simulink model "invpend_NL_PID"  (R2023b)
settings: Solver=VariableStepAuto  StartTime=0.0  StopTime=10.0  MaxStep=0.01  RelTol=1e-3
libraries: slpidlib x1
settings Model: Creator=bwang-ccny  LastModifiedBy=bwang-ccny

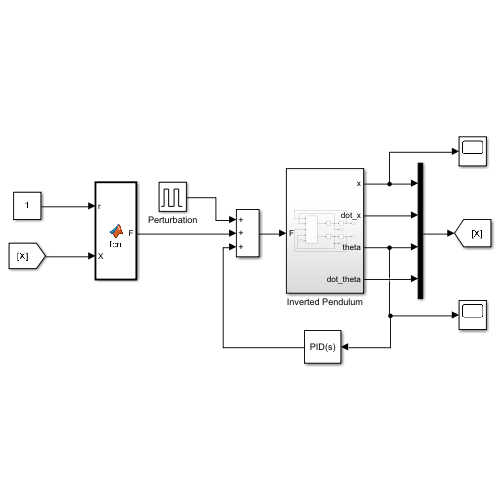
[thumbnail: Simulink's stored preview of the top-level diagram]
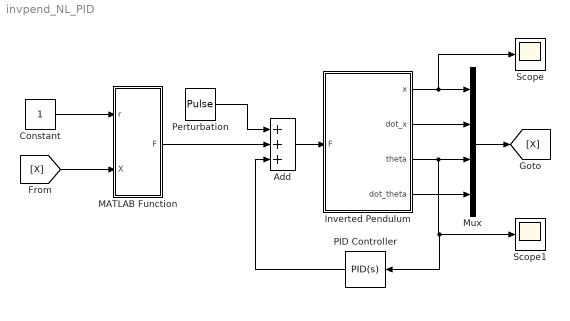
== system invpend_NL_PID ==
  Add : Sum  Inputs=+++
  Constant : Constant
  Inverted Pendulum : Subsystem
  MATLAB Function : MATLAB Function  TreatAsAtomicUnit=on
  Mux : Mux
  PID Controller : slpidlib/PID Controller  Controller=PID  Form=Parallel  TimeDomain=Continuous-time  UseExternalTs=off  SampleTime=-1  IntegratorMethod=Forward Euler  FilterMethod=Forward Euler  ControllerParametersSource=internal  P=20  I=0  UseKiTs=off  D=2  N=100  UseFilter=on  TunerSelectOption=Transfer Function Based (PID Tuner App)  InitialConditionSource=internal  InitialConditionForIntegrator=0  InitialConditionForFilter=0  DifferentiatorICPrevScaledInput=0  ExternalReset=none  TrackingMode=off  Kt=1  LimitOutput=off  SatLimitsSource=internal  UpperSaturationLimit=inf  LowerSaturationLimit=-inf  LinearizeAsGain=on  AntiWindupMode=none  Kb=1  LimitIntegrator=off  UpperIntegratorSaturationLimit=inf  LowerIntegratorSaturationLimit=-inf  POutMin=[]  POutMax=[]  IOutMin=[]  IOutMax=[]  DOutMin=[]  DOutMax=[]  NOutMin=[]  NOutMax=[]  SumOutMin=[]  SumOutMax=[]  SaturationOutMin=[]  SaturationOutMax=[]  PParamMin=[]  PParamMax=[]  IParamMin=[]  IParamMax=[]  DParamMin=[]  DParamMax=[]  NParamMin=[]  NParamMax=[]  KbParamMin=[]  KbParamMax=[]  KtParamMin=[]  KtParamMax=[]  KbOutMin=[]  KbOutMax=[]  KtOutMin=[]  KtOutMax=[]  IntegratorOutMin=[]  IntegratorOutMax=[]  FilterOutMin=[]  FilterOutMax=[]  SumI1OutMin=[]  SumI1OutMax=[]  SumI2OutMin=[]  SumI2OutMax=[]  SumI3OutMin=[]  SumI3OutMax=[]  SumI4OutMin=[]  SumI4OutMax=[]  SumDOutMin=[]  SumDOutMax=[]  DifferentiatorOutMin=[]  DifferentiatorOutMax=[]  FilterDiffOutCoefMin=[]  FilterDiffOutCoefMax=[]  ReciprocalOutMin=[]  ReciprocalOutMax=[]  SumDenOutMin=[]  SumDenOutMax=[]  SumNumOutMin=[]  SumNumOutMax=[]  DivideOutMin=[]  DivideOutMax=[]  UdiffTsProdOutMin=[]  UdiffTsProdOutMax=[]  NTsProdOutMin=[]  NTsProdOutMax=[]  UintegralTsProdOutMin=[]  UintegralTsProdOutMax=[]  UngainTsProdOutMin=[]  UngainTsProdOutMax=[]  ClampingZeroOutDataTypeStr=Inherit: Inherit via back propagation  ClampingZeroOutMin=[]  ClampingZeroOutMax=[]  FilterDenConstantOutDataTypeStr=Inherit: Inherit via back propagation  FilterDenConstantOutMin=[]  FilterDenConstantOutMax=[]  PCopyOutDataTypeStr=Inherit: Inherit via back propagation  PCopyOutMin=[]  PCopyOutMax=[]  NCopyOutDataTypeStr=Inherit: Inherit via back propagation  NCopyOutMin=[]  NCopyOutMax=[]  IntegratorContinuousStateAttributes=''  IntegratorStateMustResolveToSignalObject=off  IntegratorRTWStateStorageClass=Auto  FilterContinuousStateAttributes=''  FilterStateMustResolveToSignalObject=off  FilterRTWStateStorageClass=Auto  ParallelPVariant=InternalParameters  IdealPVariant=Disabled  IVariant=InternalParameters  DVariant=InternalParameters  IntegratorVariant=Continuous  SatVariant=Disabled  AWVariant=Passthrough  PCopyVariant=Disabled  TRVariant=Disabled  FdbkBlocksVariant=Forward  IdealPFdbkVariant=Disabled  SatFdbkVariant=Disabled  DerivativeFilterVariant=ContFilter  NVariant=InternalParameters  NCopyVariant=Disabled  FilterICVariant=InternalICsFilter  IntegratorICVariant=InternalICs  ExternalResetVariant=Disabled  TRSumVariant=Passthrough  SumFdbkVariant=Disabled  SumVariant=Sum_PID  TsampFilterVariant=InternalTs  TsampNgainVariant=Passthrough  TsampIntegralVariant=Disabled_SignalSpec  ExternalSaturationOutDataTypeStr=Inherit: Same as second input
  Perturbation : DiscretePulseGenerator  PulseType=Time based  Amplitude=10  Period=100  PulseWidth=0.1
  Scope : Scope
  Scope1 : Scope
  wires:
  Constant/1 -> MATLAB Function/1(r)
  Inverted Pendulum/1(x) -> Scope/1, Mux/1
  Inverted Pendulum/2(dot_x) -> Mux/2
  Inverted Pendulum/3(theta) -> PID Controller/1, Scope1/1, Mux/3
  Inverted Pendulum/4(dot_theta) -> Mux/4
  Mux/1 -> [X]
  [X] -> MATLAB Function/2(X)
  MATLAB Function/1(F) -> Add/2
  Add/1 -> Inverted Pendulum/1(F)
  PID Controller/1 -> Add/3
  Perturbation/1 -> Add/1

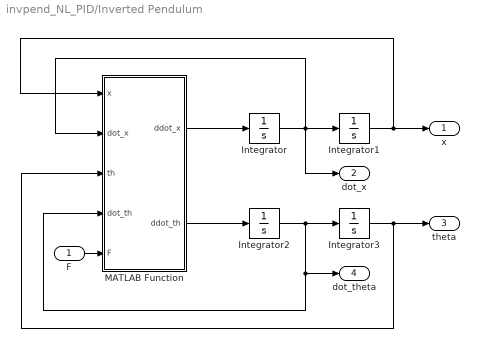
== system invpend_NL_PID/Inverted Pendulum ==
  F : Inport
  Integrator{,1..3} (4 alike) : Integrator
  MATLAB Function : MATLAB Function  TreatAsAtomicUnit=on
  x : Outport
  dot_x : Outport  Port=2
  theta : Outport  Port=3
  dot_theta : Outport  Port=4
  wires:
  Integrator/1 -> dot_x/1, MATLAB Function/2(dot_x), Integrator1/1
  MATLAB Function/2(ddot_th) -> Integrator2/1
  Integrator2/1 -> dot_theta/1, MATLAB Function/4(dot_th), Integrator3/1
  Integrator1/1 -> x/1, MATLAB Function/1(x)
  Integrator3/1 -> theta/1, MATLAB Function/3(th)
  MATLAB Function/1(ddot_x) -> Integrator/1
  F/1 -> MATLAB Function/5(F)

== matlab function invpend_NL_PID/MATLAB Function ==
  data: r input; F output; X input
function F = fcn(r, X)

x = X(1);
dot_x = X(2);
th = X(3);
dot_th = X(4);

%% LQR
% K = [-1.0000   -1.5525  -18.6696   -3.4562];

K = [0   0   0   0];
F = -K*[(x - r), dot_x, th, dot_th]';

== matlab function invpend_NL_PID/Inverted Pendulum/MATLAB Function ==
  data: x input; ddot_x output; dot_x input; th input; dot_th input; ddot_th output; F input
function [ddot_x, ddot_th] = fcn(x,dot_x,th,dot_th,F)

M = 0.5;
m = 0.2;
I = 0.006;
g = 9.8;
l = 0.3;
Q = (M + m)*(I + m*l^2) - (m*l)^2*cos(th)^2;


ddot_x = ((I + m*l^2)*(F + m*l*dot_th^2*sin(th)) - m^2*l^2*g*cos(th)*sin(th))/Q;
ddot_th = (m*l*cos(th)*F + m^2*l^2*dot_th^2*sin(th)*cos(th) - (M + m)*m*l*g*sin(th))/(-Q);
